simulink model "VoltageSourceInverter"  (R2013a)
settings: Solver=ode23tb  StartTime=5  StopTime=10  FixedStep=10^-3  MaxStep=10^-2  RelTol=1e-2
undefined symbols (not defined in the file): C, k_ic, k_iv, k_pc, k_pv, L, m_p, n_q, R_l, V_n, w, w_c, W_n
libraries: powerlib x29, PartTransformation x4, powerlib_meascontrol x1
settings Model: Creator=Elad  LastModifiedBy=USER
settings DataIOCC: SignalLoggingSaveFormat=ModelDataLogs
settings DebuggingCC: MultiTaskDSMMsg=warning  MultiTaskCondExecSysMsg=none  StateNameClashWarn=none  StrictBusMsg=None
settings RTWCC: IncludeERTFirstTime=on

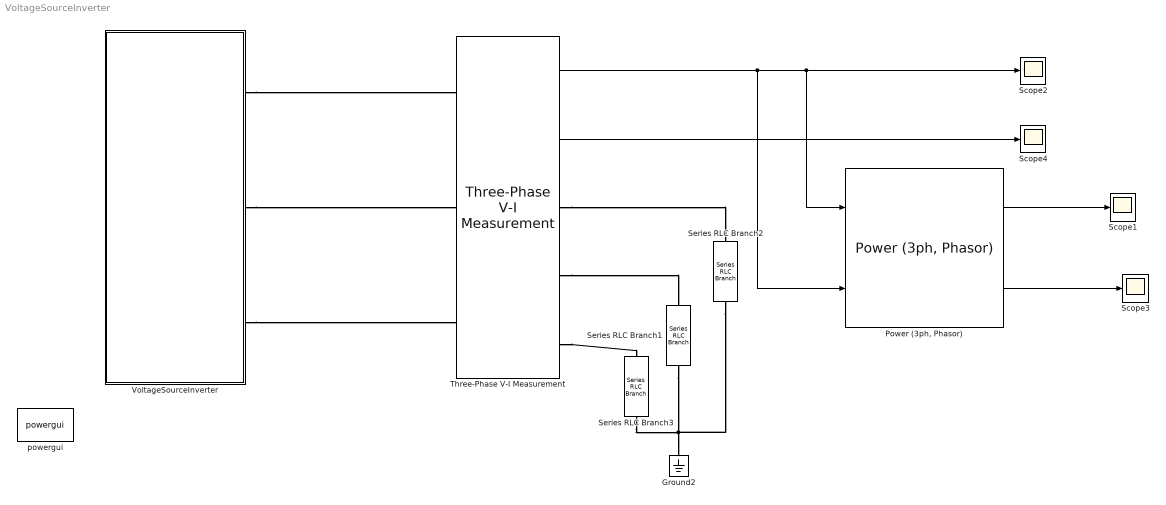
== system VoltageSourceInverter ==
  Ground2 : powerlib/Elements/Ground  LConnTagsString=a
  "Power (3ph, Phasor)" : powerlib_meascontrol/Measurements/Power (3ph, Phasor)
  Scope{1..4} (4 alike) : Scope
      Scope1 settings: TimeRange=5  YMin=5.9e+13  YMax=7.9e+13
      Scope2 settings: TimeRange=5  YMin=-8e+06  YMax=8e+06
      Scope3 settings: TimeRange=5  YMin=-225  YMax=225  SaveName=ScopeData3
      Scope4 settings: TimeRange=5  YMin=-2000  YMax=2000  SaveName=ScopeData4
  Series RLC Branch1 : powerlib/Elements/Series RLC Branch  LConnTagsString=__new0  RConnTagsString=__new0  BranchType=R  Resistance=R_l  Inductance=1e-3  SetiL0=off  InitialCurrent=0  Capacitance=1e-6  Setx0=off  InitialVoltage=0  Measurements=None
  Series RLC Branch2 : powerlib/Elements/Series RLC Branch  LConnTagsString=__new0  RConnTagsString=__new0  BranchType=R  Resistance=R_l  Inductance=1e-3  SetiL0=off  InitialCurrent=0  Capacitance=1e-6  Setx0=off  InitialVoltage=0  Measurements=None
  Series RLC Branch3 : powerlib/Elements/Series RLC Branch  LConnTagsString=__new0  RConnTagsString=__new0  BranchType=R  Resistance=R_l  Inductance=1e-3  SetiL0=off  InitialCurrent=0  Capacitance=1e-6  Setx0=off  InitialVoltage=0  Measurements=None
  Three-Phase V-I Measurement : powerlib/Measurements/Three-Phase V-I Measurement  VoltageMeasurement=phase-to-ground  SetLabelV=off  LabelV=Vabc  Vpu=off  VpuLL=off  CurrentMeasurement=yes  SetLabelI=off  LabelI=Iabc  Ipu=off  Pbase=100e6  Vbase=500e3  OutputType=Complex  PhasorSimulation=off  PSBequivalent=0
  VoltageSourceInverter : Subsystem
  powergui : powerlib/powergui  Priority=1  SimulationMode=Continuous  SolverType=Tustin  SampleTime=50e-6  frequency=60  SPID=off  DisableSnubberDevices=off  DisableRonSwitches=off  DisableVfSwitches=off  SwTol=0  Interpol=off  DisplayEquations=off  frequencyindice=0  Pbase=100e6  ErrMax=1e-4  Iterations=50  UnitsV=kV  UnitsW=MW  FunctionMessages=off  echomessages=off  HookPort=off  EnableUseOfTLC=off  x0status=blocks  RestoreLinks=warning  ResistiveCurrentMeasurement=off  Frange=[0:2:500]  Ylog=off  Xlog=on  ShowGrid=off  save=off  variable=ZData  ZoomFFT=off  StartTime=0.0  cycles=1  DisplayStyle=1  fundamental=60  FreqAxis=off  MaxFrequency=1000  frequencyindicesteady=1  RmsSteady=1  display=off  Ts=0  methode=off
  wires:
  "Power (3ph, Phasor)"/1 -> Scope1/1
  "Power (3ph, Phasor)"/2 -> Scope3/1
  Three-Phase V-I Measurement/1 -> "Power (3ph, Phasor)"/2, "Power (3ph, Phasor)"/1, Scope2/1
  Three-Phase V-I Measurement/2 -> Scope4/1
  connections:
  Series RLC Branch3/RConn1 -- Series RLC Branch2/RConn1 -- Ground2/LConn1 -- Series RLC Branch1/RConn1
  VoltageSourceInverter/RConn1 -- Three-Phase V-I Measurement/LConn1
  VoltageSourceInverter/RConn2 -- Three-Phase V-I Measurement/LConn2
  VoltageSourceInverter/RConn3 -- Three-Phase V-I Measurement/LConn3
  Three-Phase V-I Measurement/RConn3 -- Series RLC Branch3/LConn1
  Three-Phase V-I Measurement/RConn2 -- Series RLC Branch1/LConn1
  Three-Phase V-I Measurement/RConn1 -- Series RLC Branch2/LConn1

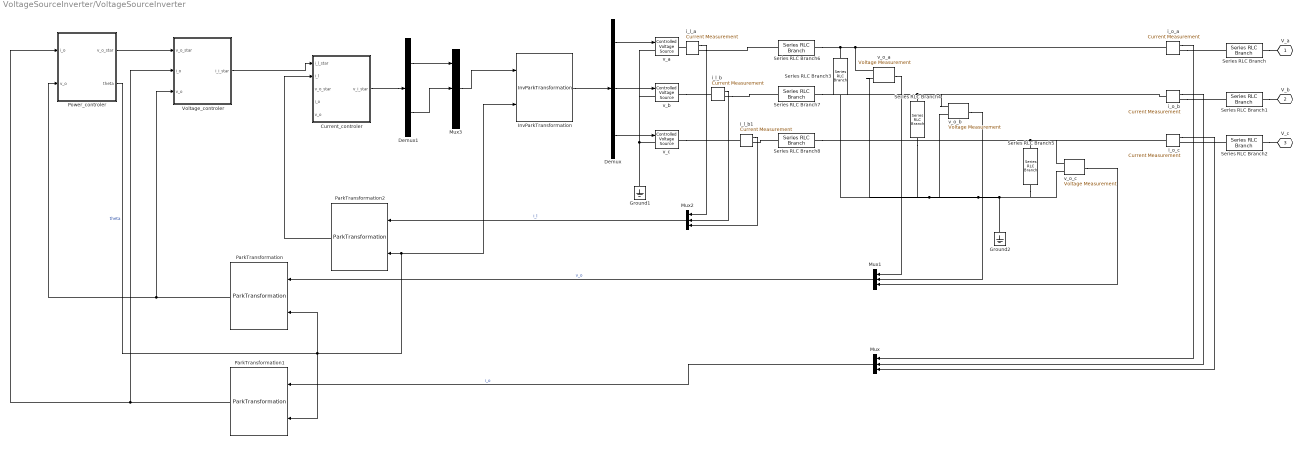
== system VoltageSourceInverter/VoltageSourceInverter ==
  Current_controler : Subsystem
  Demux : Demux  Outputs=3
  Demux1 : Demux  Outputs=2
  Ground1 : powerlib/Elements/Ground  LConnTagsString=a
  Ground2 : powerlib/Elements/Ground  LConnTagsString=a
  InvParkTransformation : PartTransformation/InvParkTransformation
  Mux{,1..3} (4 alike) : Mux  Inputs=3
  ParkTransformation : PartTransformation/ParkTransformation
  ParkTransformation1 : PartTransformation/ParkTransformation
  ParkTransformation2 : PartTransformation/ParkTransformation
  Power_controler : Subsystem
  Series RLC Branch : powerlib/Elements/Series RLC Branch  LConnTagsString=__new0  RConnTagsString=__new0  BranchType=L  Resistance=1  Inductance=1e-3  SetiL0=off  InitialCurrent=0  Capacitance=1e-6  Setx0=off  InitialVoltage=0  Measurements=None
  Series RLC Branch1 : powerlib/Elements/Series RLC Branch  LConnTagsString=__new0  RConnTagsString=__new0  BranchType=L  Resistance=1  Inductance=1e-3  SetiL0=off  InitialCurrent=0  Capacitance=1e-6  Setx0=off  InitialVoltage=0  Measurements=None
  Series RLC Branch2 : powerlib/Elements/Series RLC Branch  LConnTagsString=__new0  RConnTagsString=__new0  BranchType=L  Resistance=1  Inductance=1e-3  SetiL0=off  InitialCurrent=0  Capacitance=1e-6  Setx0=off  InitialVoltage=0  Measurements=None
  Series RLC Branch3 : powerlib/Elements/Series RLC Branch  LConnTagsString=__new0  RConnTagsString=__new0  BranchType=C  Resistance=1  Inductance=1e-3  SetiL0=off  InitialCurrent=0  Capacitance=C  Setx0=off  InitialVoltage=0  Measurements=None
  Series RLC Branch4 : powerlib/Elements/Series RLC Branch  LConnTagsString=__new0  RConnTagsString=__new0  BranchType=C  Resistance=1  Inductance=1e-3  SetiL0=off  InitialCurrent=0  Capacitance=C  Setx0=off  InitialVoltage=0  Measurements=None
  Series RLC Branch5 : powerlib/Elements/Series RLC Branch  LConnTagsString=__new0  RConnTagsString=__new0  BranchType=C  Resistance=1  Inductance=1e-3  SetiL0=off  InitialCurrent=0  Capacitance=C  Setx0=off  InitialVoltage=0  Measurements=None
  Series RLC Branch6 : powerlib/Elements/Series RLC Branch  LConnTagsString=__new0  RConnTagsString=__new0  BranchType=L  Resistance=1  Inductance=L  SetiL0=off  InitialCurrent=0  Capacitance=1e-6  Setx0=off  InitialVoltage=0  Measurements=None
  Series RLC Branch7 : powerlib/Elements/Series RLC Branch  LConnTagsString=__new0  RConnTagsString=__new0  BranchType=L  Resistance=1  Inductance=L  SetiL0=off  InitialCurrent=0  Capacitance=1e-6  Setx0=off  InitialVoltage=0  Measurements=None
  Series RLC Branch8 : powerlib/Elements/Series RLC Branch  LConnTagsString=__new0  RConnTagsString=__new0  BranchType=L  Resistance=1  Inductance=L  SetiL0=off  InitialCurrent=0  Capacitance=1e-6  Setx0=off  InitialVoltage=0  Measurements=None
  Voltage_controler : Subsystem
  i_l_a : powerlib/Measurements/Current Measurement  PhasorSimulation=off  OutputType=Complex  PSBequivalent=0
  i_l_b : powerlib/Measurements/Current Measurement  PhasorSimulation=off  OutputType=Complex  PSBequivalent=0
  i_l_b1 : powerlib/Measurements/Current Measurement  PhasorSimulation=off  OutputType=Complex  PSBequivalent=0
  i_o_a : powerlib/Measurements/Current Measurement  PhasorSimulation=off  OutputType=Complex  PSBequivalent=0
  i_o_b : powerlib/Measurements/Current Measurement  PhasorSimulation=off  OutputType=Complex  PSBequivalent=0
  i_o_c : powerlib/Measurements/Current Measurement  PhasorSimulation=off  OutputType=Complex  PSBequivalent=0
  v_a : powerlib/Electrical Sources/Controlled Voltage Source  Initialize=on  Source_Type=AC  Amplitude=0  Phase=0  Frequency=0  Measurements=None
  v_b : powerlib/Electrical Sources/Controlled Voltage Source  Initialize=on  Source_Type=AC  Amplitude=0  Phase=0  Frequency=0  Measurements=None
  v_c : powerlib/Electrical Sources/Controlled Voltage Source  Initialize=on  Source_Type=AC  Amplitude=0  Phase=0  Frequency=0  Measurements=None
  v_o_a : powerlib/Measurements/Voltage Measurement  PhasorSimulation=off  OutputType=Complex  PSBequivalent=0
  v_o_b : powerlib/Measurements/Voltage Measurement  PhasorSimulation=off  OutputType=Complex  PSBequivalent=0
  v_o_c : powerlib/Measurements/Voltage Measurement  PhasorSimulation=off  OutputType=Complex  PSBequivalent=0
  V_a : PMIOPort  Tag=PMCPort  Port=1  Side=Right
  V_b : PMIOPort  Tag=PMCPort  Port=2  Side=Right
  V_c : PMIOPort  Tag=PMCPort  Port=3  Side=Right
  wires:
  i_o_a/1 -> Mux/1
  i_o_b/1 -> Mux/2
  i_o_c/1 -> Mux/3
  v_o_a/1 -> Mux1/1
  v_o_b/1 -> Mux1/2
  v_o_c/1 -> Mux1/3
  Demux/1 -> v_a/1
  Demux/2 -> v_b/1
  Demux/3 -> v_c/1
  i_l_a/1 -> Mux2/1
  i_l_b/1 -> Mux2/2
  i_l_b1/1 -> Mux2/3
  Mux2/1 -> ParkTransformation2/1  "i_l"
  Voltage_controler/1(i_i_star) -> Current_controler/1(i_l_star)
  Power_controler/1(v_o_star) -> Voltage_controler/1(v_o_star)
  Mux1/1 -> ParkTransformation/1  "v_o"
  ParkTransformation/1 -> Power_controler/2(v_o), Voltage_controler/3(v_o)
  Mux/1 -> ParkTransformation1/1  "i_o"
  ParkTransformation1/1 -> Voltage_controler/2(i_o), Power_controler/1(i_o)
  Power_controler/2(theta) -> ParkTransformation/2, InvParkTransformation/2, ParkTransformation2/2, ParkTransformation1/2  "theta"
  ParkTransformation2/1 -> Current_controler/2(i_l)
  InvParkTransformation/1 -> Demux/1
  Current_controler/1(v_i_star) -> Demux1/1
  Mux3/1 -> InvParkTransformation/1
  Demux1/1 -> Mux3/1
  Demux1/2 -> Mux3/2
  connections:
  Series RLC Branch2/RConn1 -- V_c/RConn1
  Series RLC Branch1/RConn1 -- V_b/RConn1
  Series RLC Branch/RConn1 -- V_a/RConn1
  Series RLC Branch8/RConn1 -- v_o_c/LConn1 -- i_o_c/LConn1 -- Series RLC Branch5/LConn1
  Series RLC Branch7/RConn1 -- v_o_b/LConn1 -- i_o_b/LConn1 -- Series RLC Branch4/LConn1
  Ground2/LConn1 -- Series RLC Branch5/RConn1 -- v_o_c/LConn2 -- Series RLC Branch3/RConn1 -- v_o_a/LConn2 -- Series RLC Branch4/RConn1 -- v_o_b/LConn2
  i_o_a/LConn1 -- v_o_a/LConn1 -- Series RLC Branch3/LConn1 -- Series RLC Branch6/RConn1
  i_o_a/RConn1 -- Series RLC Branch/LConn1
  i_o_b/RConn1 -- Series RLC Branch1/LConn1
  Series RLC Branch2/LConn1 -- i_o_c/RConn1
  v_c/LConn1 -- v_a/LConn1 -- v_b/LConn1 -- Ground1/LConn1
  v_a/RConn1 -- i_l_a/LConn1
  i_l_a/RConn1 -- Series RLC Branch6/LConn1
  v_b/RConn1 -- i_l_b/LConn1
  i_l_b/RConn1 -- Series RLC Branch7/LConn1
  v_c/RConn1 -- i_l_b1/LConn1
  i_l_b1/RConn1 -- Series RLC Branch8/LConn1

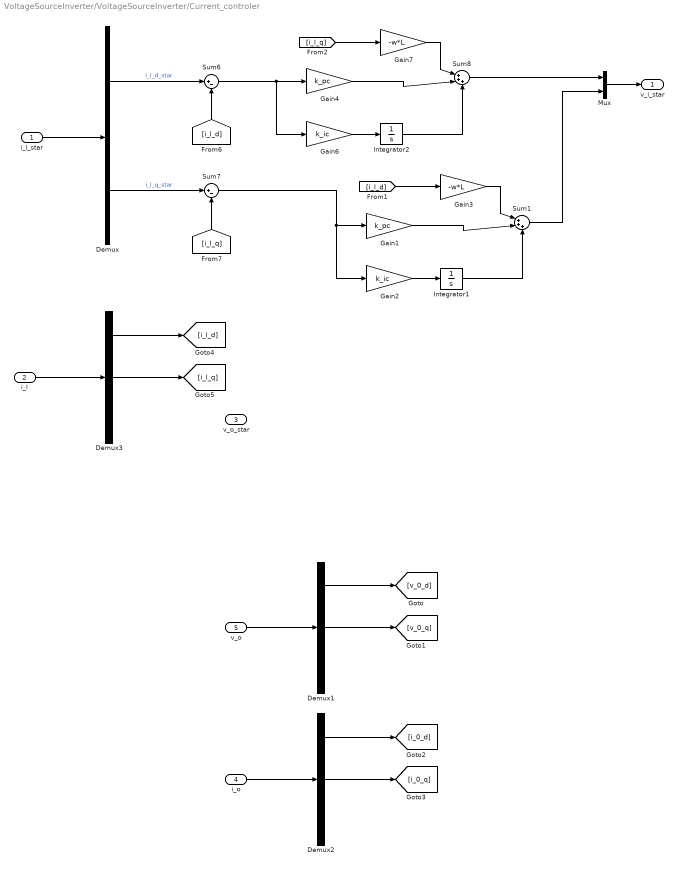
== system VoltageSourceInverter/VoltageSourceInverter/Current_controler ==
  i_l_star : Inport
  i_l : Inport  Port=2
  v_o_star : Inport  Port=3
  i_o : Inport  Port=4
  v_o : Inport  Port=5
  Demux : Demux  Outputs=2
  Demux1 : Demux  Outputs=3
  Demux2 : Demux  Outputs=3
  Demux3 : Demux  Outputs=3
  Gain1 : Gain  Gain=k_pc
  Gain2 : Gain  Gain=k_ic
  Gain3 : Gain  Gain=-w*L
  Gain4 : Gain  Gain=k_pc
  Gain6 : Gain  Gain=k_ic
  Gain7 : Gain  Gain=-w*L
  Integrator1 : Integrator
  Integrator2 : Integrator
  Mux : Mux  Inputs=2
  Sum1 : Sum  Inputs=|+++
  Sum6 : Sum  Inputs=|+-
  Sum7 : Sum  Inputs=|+-
  Sum8 : Sum  Inputs=|+++
  v_i_star : Outport
  wires:
  v_o/1 -> Demux1/1
  Demux1/1 -> [v_0_d]
  Demux1/2 -> [v_0_q]
  i_o/1 -> Demux2/1
  Demux2/1 -> [i_0_d]
  Demux2/2 -> [i_0_q]
  i_l_star/1 -> Demux/1
  Demux/1 -> Sum6/1  "i_l_d_star"
  Demux/2 -> Sum7/1  "i_l_q_star"
  i_l/1 -> Demux3/1
  Demux3/1 -> [i_l_d]
  Demux3/2 -> [i_l_q]
  [i_l_q] -> Sum7/2
  [i_l_d] -> Sum6/2
  Sum6/1 -> Gain6/1, Gain4/1
  Gain6/1 -> Integrator2/1
  Gain4/1 -> Sum8/2
  Integrator2/1 -> Sum8/3
  Gain7/1 -> Sum8/1
  [i_l_q] -> Gain7/1
  Sum7/1 -> Gain2/1, Gain1/1
  Gain2/1 -> Integrator1/1
  Gain1/1 -> Sum1/2
  Integrator1/1 -> Sum1/3
  Gain3/1 -> Sum1/1
  [i_l_d] -> Gain3/1
  Sum8/1 -> Mux/1
  Sum1/1 -> Mux/2
  Mux/1 -> v_i_star/1

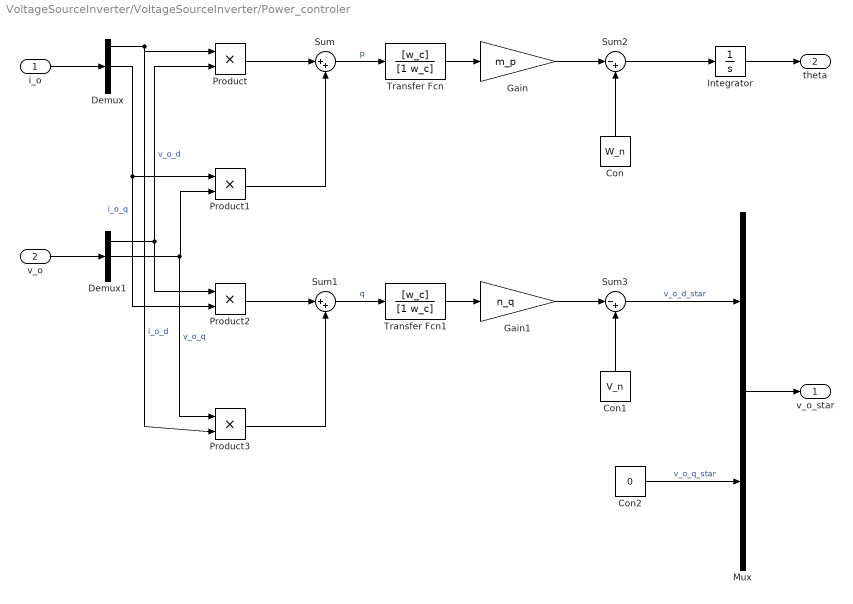
== system VoltageSourceInverter/VoltageSourceInverter/Power_controler ==
  i_o : Inport
  v_o : Inport  Port=2
  Con : Constant  Value=W_n
  Con1 : Constant  Value=V_n
  Con2 : Constant  Value=0
  Demux : Demux  Outputs=3
  Demux1 : Demux  Outputs=3
  Gain : Gain  Gain=m_p
  Gain1 : Gain  Gain=n_q
  Integrator : Integrator
  Mux : Mux  Inputs=2
  Product{,1..3} (4 alike) : Product
  Sum : Sum  Inputs=|++
  Sum1 : Sum  Inputs=|++
  Sum2 : Sum  Inputs=|-+
  Sum3 : Sum  Inputs=|-+
  Transfer Fcn : TransferFcn  Numerator=[w_c]  Denominator=[1 w_c]
  Transfer Fcn1 : TransferFcn  Numerator=[w_c]  Denominator=[1 w_c]
  v_o_star : Outport
  theta : Outport  Port=2
  wires:
  i_o/1 -> Demux/1
  v_o/1 -> Demux1/1
  Demux/1 -> Product3/2, Product/1  "i_o_d"
  Demux1/1 -> Product2/1, Product/2  "v_o_d"
  Demux/2 -> Product2/2, Product1/1  "i_o_q"
  Demux1/2 -> Product3/1, Product1/2  "v_o_q"
  Product/1 -> Sum/1
  Product1/1 -> Sum/2
  Product2/1 -> Sum1/1
  Product3/1 -> Sum1/2
  Sum/1 -> Transfer Fcn/1  "p"
  Sum1/1 -> Transfer Fcn1/1  "q"
  Transfer Fcn/1 -> Gain/1
  Transfer Fcn1/1 -> Gain1/1
  Gain/1 -> Sum2/1
  Gain1/1 -> Sum3/1
  Con/1 -> Sum2/2
  Con1/1 -> Sum3/2
  Sum2/1 -> Integrator/1
  Sum3/1 -> Mux/1  "v_o_d_star"
  Con2/1 -> Mux/2  "v_o_q_star"
  Mux/1 -> v_o_star/1
  Integrator/1 -> theta/1

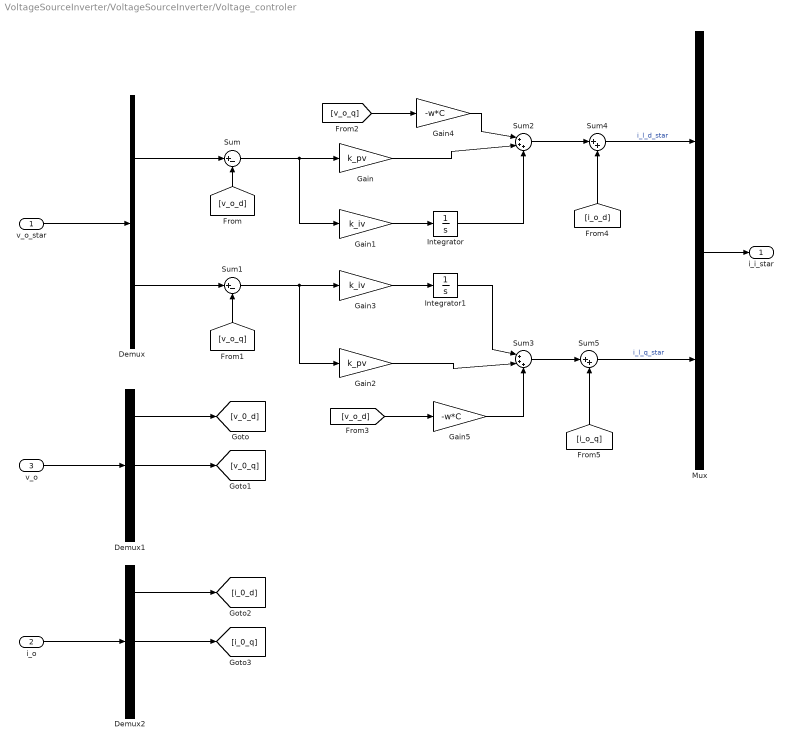
== system VoltageSourceInverter/VoltageSourceInverter/Voltage_controler ==
  v_o_star : Inport
  i_o : Inport  Port=2
  v_o : Inport  Port=3
  Demux : Demux  Outputs=2
  Demux1 : Demux  Outputs=3
  Demux2 : Demux  Outputs=3
  Gain : Gain  Gain=k_pv
  Gain1 : Gain  Gain=k_iv
  Gain2 : Gain  Gain=k_pv
  Gain3 : Gain  Gain=k_iv
  Gain4 : Gain  Gain=-w*C
  Gain5 : Gain  Gain=-w*C
  Integrator : Integrator
  Integrator1 : Integrator
  Mux : Mux  Inputs=2
  Sum : Sum  Inputs=|+-
  Sum1 : Sum  Inputs=|+-
  Sum2 : Sum  Inputs=|+++
  Sum3 : Sum  Inputs=|+++
  Sum4 : Sum  Inputs=|++
  Sum5 : Sum  Inputs=|++
  i_i_star : Outport
  wires:
  v_o_star/1 -> Demux/1
  v_o/1 -> Demux1/1
  Demux/1 -> Sum/1
  Demux1/1 -> [v_0_d]
  Demux1/2 -> [v_0_q]
  [v_o_d] -> Sum/2
  Demux/2 -> Sum1/1
  [v_o_q] -> Sum1/2
  Sum/1 -> Gain1/1, Gain/1
  Gain1/1 -> Integrator/1
  Sum1/1 -> Gain2/1, Gain3/1
  Gain3/1 -> Integrator1/1
  Integrator/1 -> Sum2/3
  Gain/1 -> Sum2/2
  Gain4/1 -> Sum2/1
  [v_o_q] -> Gain4/1
  Integrator1/1 -> Sum3/1
  Gain2/1 -> Sum3/2
  Gain5/1 -> Sum3/3
  [v_o_d] -> Gain5/1
  i_o/1 -> Demux2/1
  Demux2/1 -> [i_0_d]
  Demux2/2 -> [i_0_q]
  Sum2/1 -> Sum4/1
  [i_o_d] -> Sum4/2
  Sum3/1 -> Sum5/1
  [i_o_q] -> Sum5/2
  Sum4/1 -> Mux/1  "i_l_d_star"
  Sum5/1 -> Mux/2  "i_l_q_star"
  Mux/1 -> i_i_star/1
